simulink model "gm_LIF_Neuron_Model"  (R2023b)
settings: Solver=FixedStepAuto  StartTime=0.0  StopTime=0.5  FixedStep=h  RelTol=1e-3
undefined symbols (not defined in the file or in its folder): E_e, E_i, g_lut, h, Rm, tao_m, Vo
libraries: hdlsllib x3
settings Model: Creator=Sertan  LastModifiedBy=Sertan
settings OptimizationCC: BlockReduction=off  ConditionallyExecuteInputs=off
settings DebuggingCC: InheritedTsInSrcMsg=none

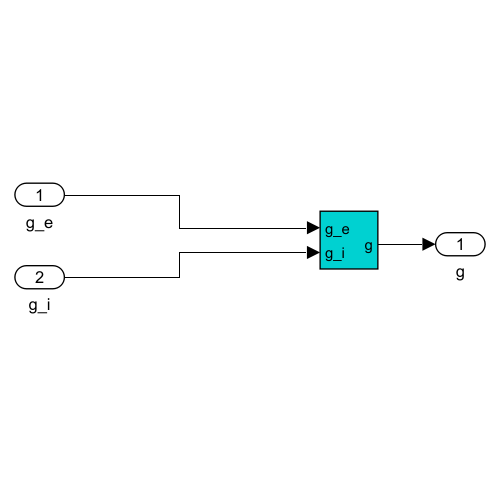
[thumbnail: Simulink's stored preview of the top-level diagram]
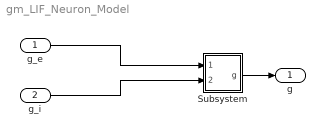
== system gm_LIF_Neuron_Model ==
  g_e : Inport  OutDataTypeStr=fixdt(1, 16, 8)  PortDimensions=1  SampleTime=0.0001
  g_i : Inport  Port=2  OutDataTypeStr=fixdt(1, 16, 8)  PortDimensions=1  SampleTime=0.0001
  Subsystem : Subsystem
  g : Outport  SampleTime=0.0001  VectorParamsAs1DForOutWhenUnconnected=off
  wires:
  g_e/1 -> Subsystem/1(g_e)
  g_i/1 -> Subsystem/2(g_i)
  Subsystem/1(g) -> g/1

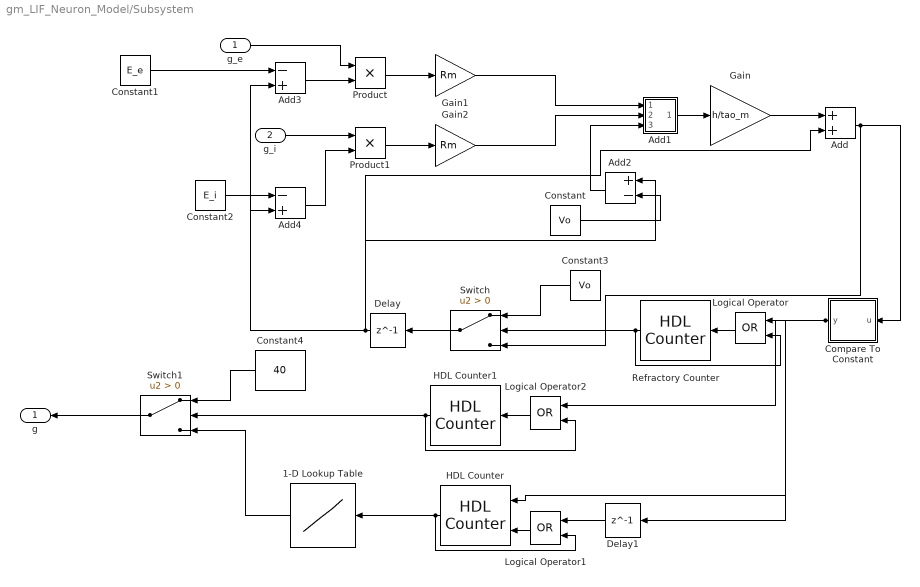
== system gm_LIF_Neuron_Model/Subsystem ==
  g_e : Inport  OutDataTypeStr=fixdt(1, 16, 8)  PortDimensions=1  SampleTime=0.0001
  g_i : Inport  Port=2  OutDataTypeStr=fixdt(1, 16, 8)  PortDimensions=1  SampleTime=0.0001
  1-D Lookup Table : Lookup_n-D  NumberOfTableDimensions=1  LookupTableObject=''  BreakpointsForDimension1=[0:201]  BreakpointsForDimension1FirstPoint=10  BreakpointsForDimension2FirstPoint=10  BreakpointsForDimension1Spacing=12  BreakpointsForDimension2Spacing=12  BreakpointsForDimension1DataTypeStr=Inherit: Inherit from 'Breakpoint data'  IndexSearchMethod=Evenly spaced points  Table=g_lut  InterpMethod=Flat  DiagnosticForOutOfRangeInput=Error  InternalRulePriority=Speed  OutDataTypeStr=fixdt(1,16,8)  RndMeth=Simplest
  Add : Sum
  Add1 : Subsystem
  Add2 : Sum  Inputs=+-
  Add3 : Sum  Inputs=-+
  Add4 : Sum  Inputs=-+
  Compare To Constant : Subsystem  mask(Compare To Constant){relop=>=, const=double(-50), OutDataTypeStr=boolean, ZeroCross=on}
      mask prompts: relop "Simulink:masks:Operator_MP"; const "Simulink:masks:ConstantValue_MP"; OutDataTypeStr "Simulink:masks:OutputDataType_MP"; ZeroCross "Simulink:masks:EnableZerocrossingDetection_MP"
      mask help: Simulink:masks:CompareToConstant_MD
      mask init:
      | OutDataTypeStr = 'boolean';
      | ZeroCross = 'on';
      | blkName = 'LIF_Neuron_Model/Subsystem/Compare\nTo Constant';
      | const = double(-50);
      | const_str = 'V_thr';
      | const_val = [];
      | relop = '>=';
      | setValue = 'boolean';
      | str = '>= V_thr';
      mask TypeOptions relop: == | ~= | < | <= | >= | >
      mask TypeOptions OutDataTypeStr: Simulink:masks:uint8 | Simulink:masks:boolean
      mask Callback ZeroCross: sl('zeroCrossEnable', gcbh);
      mask Display: disp(str)
  Constant : Constant  Value=Vo  OutDataTypeStr=fixdt(1,16,8)
  Constant1 : Constant  Value=E_e  OutDataTypeStr=fixdt(1,16,8)
  Constant2 : Constant  Value=E_i  OutDataTypeStr=fixdt(1,16,8)
  Constant3 : Constant  Value=Vo  OutDataTypeStr=fixdt(1,16,8)
  Constant4 : Constant  Value=40  OutDataTypeStr=fixdt(1,16,8)
  Delay : Delay  DelayLength=1  InitialCondition=Vo
  Delay1 : Delay  DelayLength=1  InitialCondition=0
  Gain : Gain  Gain=h/tao_m  OutDataTypeStr=fixdt(1,16,8)
  Gain1 : Gain  Gain=Rm
  Gain2 : Gain  Gain=Rm
  HDL Counter : hdlsllib/Sources/HDL Counter  CountType=Count limited  CountInit=0  CountStep=1  CountMax=length(g_lut)-1  CountFromType=Initial value  CountFrom=0  CountResetPort=on  CountLoadPort=off  CountEnbPort=on  CountDirPort=off  CountHitOutputPort=off  CountDataType=Unsigned  CountWordLen=8  CountFracLen=0  CountSampTime=1
  HDL Counter1 : hdlsllib/Sources/HDL Counter  CountType=Count limited  CountInit=0  CountStep=1  CountMax=2  CountFromType=Initial value  CountFrom=0  CountResetPort=off  CountLoadPort=off  CountEnbPort=on  CountDirPort=off  CountHitOutputPort=off  CountDataType=Unsigned  CountWordLen=8  CountFracLen=0  CountSampTime=1
  Logical Operator : Logic  Operator=OR  AllPortsSameDT=off  OutDataTypeStr=boolean
  Logical Operator1 : Logic  Operator=OR  AllPortsSameDT=off  OutDataTypeStr=boolean
  Logical Operator2 : Logic  Operator=OR  AllPortsSameDT=off  OutDataTypeStr=boolean
  Product : Product
  Product1 : Product
  Refractory Counter : hdlsllib/Sources/HDL Counter  CountType=Count limited  CountInit=0  CountStep=1  CountMax=r_time  CountFromType=Initial value  CountFrom=0  CountResetPort=off  CountLoadPort=off  CountEnbPort=on  CountDirPort=off  CountHitOutputPort=off  CountDataType=Unsigned  CountWordLen=8  CountFracLen=0  CountSampTime=1
  Switch : Switch  Criteria=u2 > Threshold  SaturateOnIntegerOverflow=off  InputSameDT=off
  Switch1 : Switch  Criteria=u2 > Threshold  OutDataTypeStr=fixdt(1,16,8)  SaturateOnIntegerOverflow=off  InputSameDT=off
  g : Outport  SampleTime=0.0001  VectorParamsAs1DForOutWhenUnconnected=off
  wires:
  g_e/1 -> Product/1
  g_i/1 -> Product1/1
  1-D Lookup Table/1 -> Switch1/3
  Add/1 -> Switch/3, Compare To Constant/1(u)
  Add1/1(Out1) -> Gain/1
  Add2/1 -> Add1/3(In3)
  Add3/1 -> Product/2
  Add4/1 -> Product1/2
  Compare To Constant/1(y) -> Logical Operator2/1, Logical Operator/1, Delay1/1, HDL Counter/1
  Constant/1 -> Add2/2
  Constant1/1 -> Add3/1
  Constant2/1 -> Add4/1
  Constant3/1 -> Switch/1
  Constant4/1 -> Switch1/1
  Delay/1 -> Add4/2, Add3/2, Add2/1, Add/2
  Delay1/1 -> Logical Operator1/1
  Gain/1 -> Add/1
  Gain1/1 -> Add1/1(In1)
  Gain2/1 -> Add1/2(In2)
  HDL Counter/1 -> Logical Operator1/2, 1-D Lookup Table/1
  HDL Counter1/1 -> Switch1/2, Logical Operator2/2
  Logical Operator/1 -> Refractory Counter/1
  Logical Operator1/1 -> HDL Counter/2
  Logical Operator2/1 -> HDL Counter1/1
  Product/1 -> Gain1/1
  Product1/1 -> Gain2/1
  Refractory Counter/1 -> Switch/2, Logical Operator/2
  Switch/1 -> Delay/1
  Switch1/1 -> g/1

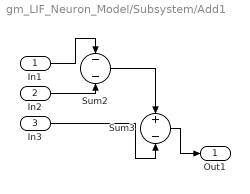
== system gm_LIF_Neuron_Model/Subsystem/Add1 ==
  In1 : Inport  OutDataTypeStr=fixdt(1,64,49)
  In2 : Inport  Port=2  OutDataTypeStr=fixdt(1,64,49)
  In3 : Inport  Port=3  OutDataTypeStr=fixdt(1,16,8)
  Sum2 : Sum  Inputs=--  OutDataTypeStr=fixdt(1,64,49)  AccumDataTypeStr=fixdt(1,64,49)
  Sum3 : Sum  Inputs=+-  OutDataTypeStr=fixdt(1,64,49)  AccumDataTypeStr=fixdt(1,64,49)
  Out1 : Outport
  wires:
  In1/1 -> Sum2/1
  In2/1 -> Sum2/2
  Sum2/1 -> Sum3/1
  In3/1 -> Sum3/2
  Sum3/1 -> Out1/1

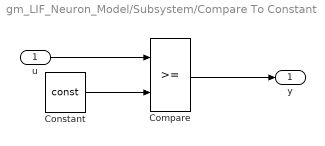
== system gm_LIF_Neuron_Model/Subsystem/Compare To Constant ==
  u : Inport  OutDataTypeStr=fixdt(1, 16, 8)  SampleTime=0.0001
  Compare : RelationalOperator  OutDataTypeStr=boolean
  Constant : Constant  DisableCoverage=on  Value=const  OutDataTypeStr=Inherit: Inherit via back propagation  SampleTime=-1
  y : Outport  SampleTime=0.0001
  wires:
  u/1 -> Compare/1
  Compare/1 -> y/1
  Constant/1 -> Compare/2
